simulink model "pll_2016a"  (R2016a)
settings: Solver=ode45  SolverMode=SingleTasking  StartTime=0.0  StopTime=1  MaxStep=1e-6  RelTol=1e-3
libraries: powerlib x20, simulink x6, powerlib_meascontrol x4
settings Model: Creator=hasee  LastModifiedBy=Junhong
settings DebuggingCC: SFUnexpectedBacktrackingDiag=error  SFNoUnconditionalDefaultTransitionDiag=error
settings GRTTargetCC: TargetLangStandard=C99 (ISO)  GeneratePreprocessorConditionals=Use local settings
settings ConfigComp: CovMetricSettings=dwe  CovHtmlReporting=off  CovSaveCumulativeToWorkspaceVar=off  CovSaveSingleToWorkspaceVar=off  CovExternalEMLEnable=on

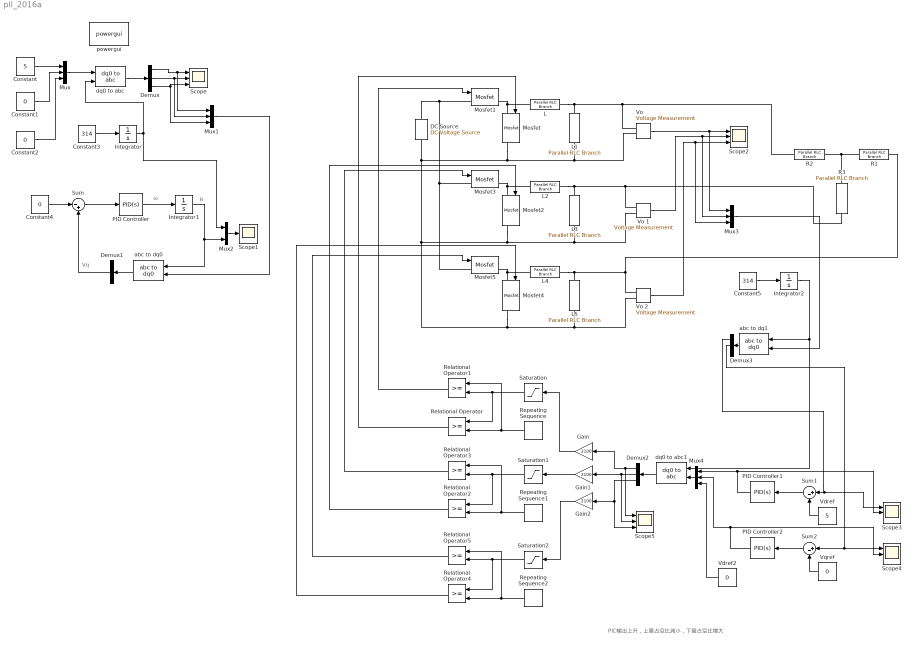
== system pll_2016a ==
  note: θ
  note: ω
  note: Vq
  note: PID输出上升，上管占空比减小，下管占空比增大
  Constant : Constant  Value=5
  Constant1 : Constant  Value=0
  Constant2 : Constant  Value=0
  Constant3 : Constant  Value=314
  Constant4 : Constant  Value=0
  Constant5 : Constant  Value=314
  DC Source : powerlib/Electrical Sources/DC Voltage Source  Amplitude=24  Measurements=None
  Demux{,1..3} (4 alike) : Demux  Outputs=3
  Gain : Gain  Gain=2100
  Gain1 : Gain  Gain=2100
  Gain2 : Gain  Gain=2100
  Integrator : Integrator
  Integrator1 : Integrator
  Integrator2 : Integrator
  L : powerlib/Elements/Parallel RLC Branch  LConnTagsString=a  RConnTagsString=__new0  BranchType=L  Resistance=1  Inductance=500e-6  SetiL0=off  InitialCurrent=0  Capacitance=1e-6  Setx0=off  InitialVoltage=0  Measurements=None
  L1 : powerlib/Elements/Parallel RLC Branch  LConnTagsString=a  RConnTagsString=__new0  BranchType=C  Resistance=0.047  Inductance=1e-3  SetiL0=off  InitialCurrent=0  Capacitance=10e-6  Setx0=off  InitialVoltage=0  Measurements=None
  L2 : powerlib/Elements/Parallel RLC Branch  LConnTagsString=a  RConnTagsString=__new0  BranchType=L  Resistance=1  Inductance=500e-6  SetiL0=off  InitialCurrent=0  Capacitance=1e-6  Setx0=off  InitialVoltage=0  Measurements=None
  L3 : powerlib/Elements/Parallel RLC Branch  LConnTagsString=a  RConnTagsString=__new0  BranchType=C  Resistance=0.047  Inductance=1e-3  SetiL0=off  InitialCurrent=0  Capacitance=10e-6  Setx0=off  InitialVoltage=0  Measurements=None
  L4 : powerlib/Elements/Parallel RLC Branch  LConnTagsString=a  RConnTagsString=__new0  BranchType=L  Resistance=1  Inductance=500e-6  SetiL0=off  InitialCurrent=0  Capacitance=1e-6  Setx0=off  InitialVoltage=0  Measurements=None
  L5 : powerlib/Elements/Parallel RLC Branch  LConnTagsString=a  RConnTagsString=__new0  BranchType=C  Resistance=0.047  Inductance=1e-3  SetiL0=off  InitialCurrent=0  Capacitance=10e-6  Setx0=off  InitialVoltage=0  Measurements=None
  Mosfet{,1..5} (6 alike) : powerlib/Power Electronics/Mosfet  Ron=0.1  Lon=0  Rd=0.01  Vfd=0  IC=0  Rs=1e5  Cs=inf  Measurements=on
  Mux{,1,3..4} (4 alike) : Mux  Inputs=3
  Mux2 : Mux  Inputs=2
  PID Controller : simulink/Continuous/PID Controller  Controller=PID  TimeDomain=Continuous-time  SampleTime=-1  IntegratorMethod=Forward Euler  FilterMethod=Forward Euler  Form=Parallel  UseFilter=on  ControllerParametersSource=internal  P=100  I=100  D=0  N=1000000  InitialConditionSource=internal  InitialConditionForIntegrator=0  InitialConditionForFilter=0  ExternalReset=none  LimitOutput=off  UpperSaturationLimit=inf  LowerSaturationLimit=-inf  LinearizeAsGain=on  AntiWindupMode=none  Kb=1  TrackingMode=off  Kt=1  PParamMin=[]  PParamMax=[]  IParamMin=[]  IParamMax=[]  DParamMin=[]  DParamMax=[]  NParamMin=[]  NParamMax=[]  KbParamMin=[]  KbParamMax=[]  KtParamMin=[]  KtParamMax=[]  POutMin=[]  POutMax=[]  IOutMin=[]  IOutMax=[]  DOutMin=[]  DOutMax=[]  NOutMin=[]  NOutMax=[]  KbOutMin=[]  KbOutMax=[]  KtOutMin=[]  KtOutMax=[]  IntegratorOutMin=[]  IntegratorOutMax=[]  FilterOutMin=[]  FilterOutMax=[]  SumOutMin=[]  SumOutMax=[]  SumI1OutMin=[]  SumI1OutMax=[]  SumI2OutMin=[]  SumI2OutMax=[]  SumI3OutMin=[]  SumI3OutMax=[]  SumDOutMin=[]  SumDOutMax=[]  SaturationOutMin=[]  SaturationOutMax=[]  IntegratorContinuousStateAttributes=''  IntegratorStateMustResolveToSignalObject=off  IntegratorRTWStateStorageClass=Auto  FilterContinuousStateAttributes=''  FilterStateMustResolveToSignalObject=off  FilterRTWStateStorageClass=Auto  DifferentiatorICPrevScaledInput=0  DifferentiatorOutMin=[]  DifferentiatorOutMax=[]
  PID Controller1 : simulink/Continuous/PID Controller  Controller=PID  TimeDomain=Continuous-time  SampleTime=-1  IntegratorMethod=Forward Euler  FilterMethod=Forward Euler  Form=Parallel  UseFilter=on  ControllerParametersSource=internal  P=1  I=1  D=0  N=1000000  InitialConditionSource=internal  InitialConditionForIntegrator=0  InitialConditionForFilter=0  ExternalReset=none  LimitOutput=off  UpperSaturationLimit=inf  LowerSaturationLimit=-inf  LinearizeAsGain=on  AntiWindupMode=none  Kb=1  TrackingMode=off  Kt=1  PParamMin=[]  PParamMax=[]  IParamMin=[]  IParamMax=[]  DParamMin=[]  DParamMax=[]  NParamMin=[]  NParamMax=[]  KbParamMin=[]  KbParamMax=[]  KtParamMin=[]  KtParamMax=[]  POutMin=[]  POutMax=[]  IOutMin=[]  IOutMax=[]  DOutMin=[]  DOutMax=[]  NOutMin=[]  NOutMax=[]  KbOutMin=[]  KbOutMax=[]  KtOutMin=[]  KtOutMax=[]  IntegratorOutMin=[]  IntegratorOutMax=[]  FilterOutMin=[]  FilterOutMax=[]  SumOutMin=[]  SumOutMax=[]  SumI1OutMin=[]  SumI1OutMax=[]  SumI2OutMin=[]  SumI2OutMax=[]  SumI3OutMin=[]  SumI3OutMax=[]  SumDOutMin=[]  SumDOutMax=[]  SaturationOutMin=[]  SaturationOutMax=[]  IntegratorContinuousStateAttributes=''  IntegratorStateMustResolveToSignalObject=off  IntegratorRTWStateStorageClass=Auto  FilterContinuousStateAttributes=''  FilterStateMustResolveToSignalObject=off  FilterRTWStateStorageClass=Auto  DifferentiatorICPrevScaledInput=0  DifferentiatorOutMin=[]  DifferentiatorOutMax=[]
  PID Controller2 : simulink/Continuous/PID Controller  Controller=PID  TimeDomain=Continuous-time  SampleTime=-1  IntegratorMethod=Forward Euler  FilterMethod=Forward Euler  Form=Parallel  UseFilter=on  ControllerParametersSource=internal  P=0  I=1  D=0  N=1000000  InitialConditionSource=internal  InitialConditionForIntegrator=0  InitialConditionForFilter=0  ExternalReset=none  LimitOutput=off  UpperSaturationLimit=inf  LowerSaturationLimit=-inf  LinearizeAsGain=on  AntiWindupMode=none  Kb=1  TrackingMode=off  Kt=1  PParamMin=[]  PParamMax=[]  IParamMin=[]  IParamMax=[]  DParamMin=[]  DParamMax=[]  NParamMin=[]  NParamMax=[]  KbParamMin=[]  KbParamMax=[]  KtParamMin=[]  KtParamMax=[]  POutMin=[]  POutMax=[]  IOutMin=[]  IOutMax=[]  DOutMin=[]  DOutMax=[]  NOutMin=[]  NOutMax=[]  KbOutMin=[]  KbOutMax=[]  KtOutMin=[]  KtOutMax=[]  IntegratorOutMin=[]  IntegratorOutMax=[]  FilterOutMin=[]  FilterOutMax=[]  SumOutMin=[]  SumOutMax=[]  SumI1OutMin=[]  SumI1OutMax=[]  SumI2OutMin=[]  SumI2OutMax=[]  SumI3OutMin=[]  SumI3OutMax=[]  SumDOutMin=[]  SumDOutMax=[]  SaturationOutMin=[]  SaturationOutMax=[]  IntegratorContinuousStateAttributes=''  IntegratorStateMustResolveToSignalObject=off  IntegratorRTWStateStorageClass=Auto  FilterContinuousStateAttributes=''  FilterStateMustResolveToSignalObject=off  FilterRTWStateStorageClass=Auto  DifferentiatorICPrevScaledInput=0  DifferentiatorOutMin=[]  DifferentiatorOutMax=[]
  R1 : powerlib/Elements/Parallel RLC Branch  LConnTagsString=a  RConnTagsString=__new0  BranchType=R  Resistance=20  Inductance=0.00033  SetiL0=off  InitialCurrent=0  Capacitance=1e-6  Setx0=off  InitialVoltage=0  Measurements=None
  R2 : powerlib/Elements/Parallel RLC Branch  LConnTagsString=a  RConnTagsString=__new0  BranchType=R  Resistance=20  Inductance=0.00033  SetiL0=off  InitialCurrent=0  Capacitance=1e-6  Setx0=off  InitialVoltage=0  Measurements=None
  R3 : powerlib/Elements/Parallel RLC Branch  LConnTagsString=a  RConnTagsString=__new0  BranchType=R  Resistance=20  Inductance=0.00033  SetiL0=off  InitialCurrent=0  Capacitance=1e-6  Setx0=off  InitialVoltage=0  Measurements=None
  Relational Operator{,1..5} (6 alike) : RelationalOperator  OutDataTypeStr=boolean
  Repeating Sequence : simulink/Sources/Repeating Sequence  rep_seq_t=[0 2.5e-5]  rep_seq_y=[-1050 1050]
  Repeating Sequence1 : simulink/Sources/Repeating Sequence  rep_seq_t=[0 2.5e-5]  rep_seq_y=[-1050 1050]
  Repeating Sequence2 : simulink/Sources/Repeating Sequence  rep_seq_t=[0 2.5e-5]  rep_seq_y=[-1050 1050]
  Saturation : Saturate  UpperLimit=1050  LowerLimit=-1050
  Saturation1 : Saturate  UpperLimit=1050  LowerLimit=-1050
  Saturation2 : Saturate  UpperLimit=1050  LowerLimit=-1050
  Scope{,2..5} (5 alike) : Scope  NumInputPorts=3
  Scope1 : Scope
  Sum : Sum  Inputs=|-+
  Sum1 : Sum  Inputs=|+-
  Sum2 : Sum  Inputs=|+-
  Vdref : Constant  Value=5
  Vdref2 : Constant  Value=0
  "Vo " : powerlib/Measurements/Voltage Measurement  PhasorSimulation=off  OutputType=Complex  PSBequivalent=0
  Vo 1 : powerlib/Measurements/Voltage Measurement  PhasorSimulation=off  OutputType=Complex  PSBequivalent=0
  Vo 2 : powerlib/Measurements/Voltage Measurement  PhasorSimulation=off  OutputType=Complex  PSBequivalent=0
  Vqref : Constant  Value=0
  abc to dq0 : powerlib_meascontrol/Transformations/abc to dq0  Alignment=Aligned with phase A axis
  abc to dq1 : powerlib_meascontrol/Transformations/abc to dq0  Alignment=Aligned with phase A axis
  dq0 to abc : powerlib_meascontrol/Transformations/dq0 to abc  Alignment=Aligned with phase A axis
  dq0 to abc1 : powerlib_meascontrol/Transformations/dq0 to abc  Alignment=Aligned with phase A axis
  powergui : powerlib/powergui  Priority=1  SimulationMode=Continuous  SolverType=Tustin/Backward Euler (TBE)  SampleTime=50e-6  frequency=60  SPID=off  DisableSnubberDevices=off  DisableRonSwitches=off  DisableVfSwitches=off  SwTol=0  DisplayEquations=off  Interpol=off  ExternalGateDelay=off  methode=off  Ts=10  FunctionMessages=off  echomessages=off  HookPort=off  EnableUseOfTLC=off  x0status=blocks  frequencyindice=0  Pbase=100e6  ErrMax=1e-4  Iterations=50  UnitsV=kV  UnitsW=MW  buscounter=0  RestoreLinks=warning  ResistiveCurrentMeasurement=off  Frange=[0:2:500]  Ylog=off  Xlog=on  ShowGrid=off  save=off  variable=ZData  structure=0  ZoomFFT=off  StartTime=0.0  cycles=1  DisplayStyle=1  fundamental=60  FreqAxis=off  MaxFrequency=1000  frequencyindicesteady=1  RmsSteady=1  display=off
  wires:
  Constant/1 -> Mux/1
  Constant1/1 -> Mux/2
  Constant2/1 -> Mux/3
  Mux/1 -> dq0 to abc/1
  dq0 to abc/1 -> Demux/1
  Demux/1 -> Mux1/1, Scope/1
  Demux/2 -> Mux1/2, Scope/2
  Demux/3 -> Mux1/3, Scope/3
  Integrator/1 -> Mux2/1, dq0 to abc/2
  Constant3/1 -> Integrator/1
  Constant4/1 -> Sum/1
  abc to dq0/1 -> Demux1/1
  Sum/1 -> PID Controller/1
  PID Controller/1 -> Integrator1/1
  Integrator1/1 -> abc to dq0/2, Mux2/2
  Mux1/1 -> abc to dq0/1
  Mux2/1 -> Scope1/1
  Demux1/2 -> Sum/2
  Vdref/1 -> Sum1/2
  Saturation/1 -> Relational Operator/1, Relational Operator1/2
  "Vo "/1 -> Mux3/1, Scope2/1
  Repeating Sequence/1 -> Relational Operator1/1, Relational Operator/2
  Relational Operator/1 -> Mosfet/1
  Relational Operator1/1 -> Mosfet1/1
  Vo 1/1 -> Mux3/2, Scope2/2
  Vo 2/1 -> Mux3/3, Scope2/3
  Integrator2/1 -> dq0 to abc1/2, abc to dq1/2
  Constant5/1 -> Integrator2/1
  Mux3/1 -> abc to dq1/1
  Saturation1/1 -> Relational Operator2/1, Relational Operator3/2
  Repeating Sequence1/1 -> Relational Operator3/1, Relational Operator2/2
  Relational Operator2/1 -> Mosfet2/1
  Relational Operator3/1 -> Mosfet3/1
  Saturation2/1 -> Relational Operator4/1, Relational Operator5/2
  Repeating Sequence2/1 -> Relational Operator5/1, Relational Operator4/2
  Relational Operator4/1 -> Mosfet4/1
  Relational Operator5/1 -> Mosfet5/1
  dq0 to abc1/1 -> Demux2/1
  abc to dq1/1 -> Demux3/1
  Mux4/1 -> dq0 to abc1/1
  PID Controller2/1 -> Mux4/2, Scope4/2
  Sum1/1 -> PID Controller1/1
  Vqref/1 -> Sum2/2
  Sum2/1 -> PID Controller2/1
  Demux3/1 -> Scope3/1, Sum1/1
  Demux3/2 -> Sum2/1, Scope4/1
  Gain/1 -> Saturation/1
  Demux2/2 -> Scope5/2, Gain1/1
  Gain1/1 -> Saturation1/1
  Demux2/3 -> Scope5/3, Gain2/1
  Gain2/1 -> Saturation2/1
  Demux2/1 -> Scope5/1, Gain/1
  Vdref2/1 -> Mux4/3
  PID Controller1/1 -> Mux4/1, Scope3/2
  connections:
  "Vo "/LConn1 -- R2/LConn1 -- L/RConn1 -- L1/LConn1
  DC Source/LConn1 -- Mosfet/RConn1 -- "Vo "/LConn2 -- L1/RConn1 -- Mosfet2/RConn1 -- L3/RConn1 -- Vo 1/LConn2 -- Mosfet4/RConn1 -- Vo 2/LConn2 -- L5/RConn1
  Mosfet/LConn1 -- Mosfet1/RConn1 -- L/LConn1
  DC Source/RConn1 -- Mosfet3/LConn1 -- Mosfet5/LConn1 -- Mosfet1/LConn1
  Mosfet2/LConn1 -- Mosfet3/RConn1 -- L2/LConn1
  Mosfet4/LConn1 -- Mosfet5/RConn1 -- L4/LConn1
  L2/RConn1 -- R3/RConn1 -- Vo 1/LConn1 -- L3/LConn1
  L4/RConn1 -- R1/RConn1 -- Vo 2/LConn1 -- L5/LConn1
  R1/LConn1 -- R3/LConn1 -- R2/RConn1
